simulink model "case_1_lead_veh_sudden_stop_25a"  (R2025b)
settings: Solver=VariableStepAuto  StartTime=0.0  StopTime=10.0  RelTol=1e-3
settings Model: Creator=admin  LastModifiedBy=admin

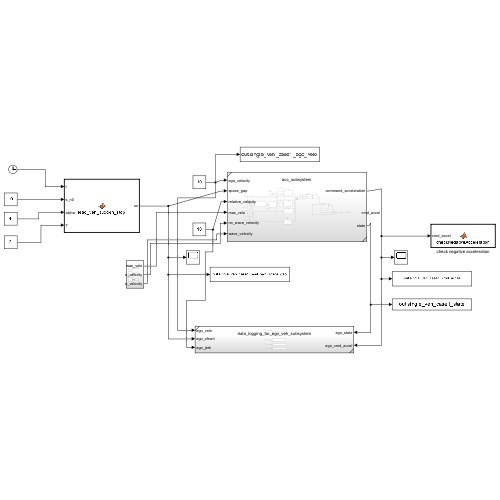
[thumbnail: Simulink's stored preview of the top-level diagram]
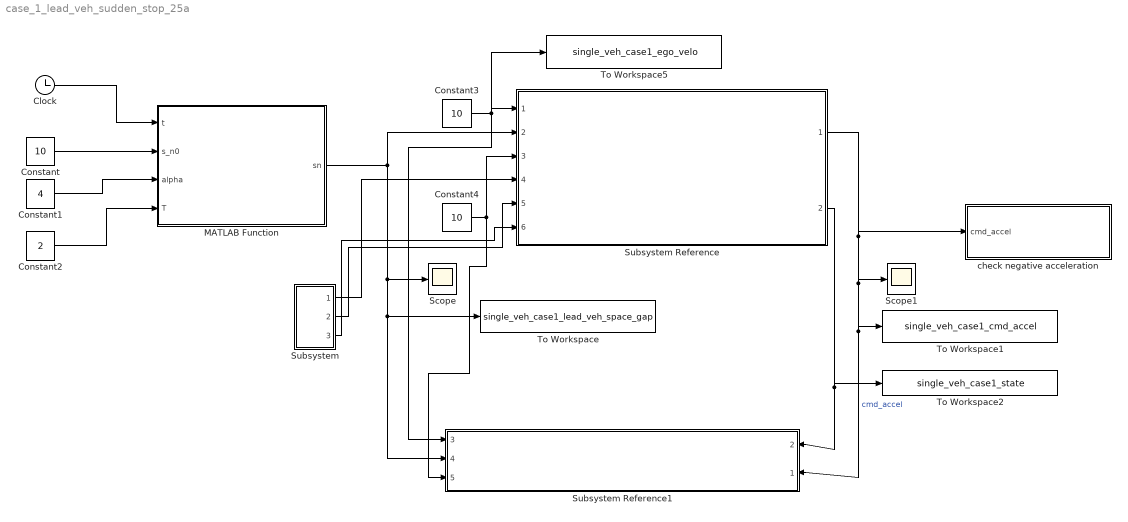
== system case_1_lead_veh_sudden_stop_25a ==
  Clock : Clock
  Constant : Constant  Value=10
  Constant1 : Constant  Value=4
  Constant2 : Constant  Value=2
  Constant3 : Constant  Value=10
  Constant4 : Constant  Value=10
  MATLAB Function : MATLAB Function  TreatAsAtomicUnit=on
  Scope : Scope
      settings: ActiveDisplayYMinimum=-2.4454295544676485  ActiveDisplayYMaximum=12.748398570532352
  Scope1 : Scope
      settings: ActiveDisplayYMinimum=-4  ActiveDisplayYMaximum=-2
  Subsystem : Subsystem
  Subsystem Reference : Subsystem  ReferencedSubsystem=acc_subsystem
  Subsystem Reference1 : Subsystem  ReferencedSubsystem=data_logging_for_ego_veh_subsystem
      settings: PortSchema="{\"entries\":[{\"content\":{\"sides\":[{\"content\":{\"connectorIds\":[\"In3\",\"In4\",\"In5\"]},\"type\":\"ConnectorPlacement.EquallySpacedRectSide\",\"uuid\":\"0b96bcaa-a470-46c9-9268-f4bd6b1035a8\"},{\"content\":{\"connectorIds\":[\"In2\",\"In1\"],\"side\":\"RIGHT\"},\"type\":\"ConnectorPlacement.EquallySpacedRectSide\",\"uuid\":\"8e49005a-1e53-4e76-b163-50df0eb9f2cc\"},{\"content\":{\"side\":\"TOP\"},\"type\":\"ConnectorPlacement.EquallySpacedRectSide\",\"uuid\":\"3ff4af65-efca-4a64-9b7f-f479498e89e2\"}]},\"type\":\"ConnectorPlacement.EquallySpacedConnector\",\"uuid\":\"f10caef7-9599-4d5c-a8fd-3eb49f6fcaa8\"}],\"packageUris\":[\"http://schema.mathworks.com/mf0/Connector/R2020b\"],\"version\":\"1.0\"}"
  To Workspace : ToWorkspace  VariableName=single_veh_case1_lead_veh_space_gap  SaveFormat=Structure With Time  SampleTime=-1
  To Workspace1 : ToWorkspace  VariableName=single_veh_case1_cmd_accel  SaveFormat=Structure With Time  SampleTime=-1
  To Workspace2 : ToWorkspace  VariableName=single_veh_case1_state  SaveFormat=Structure With Time  SampleTime=-1
  To Workspace5 : ToWorkspace  VariableName=single_veh_case1_ego_velo  SaveFormat=Structure With Time  SampleTime=-1
  check negative acceleration : MATLAB Function  TreatAsAtomicUnit=on
  wires:
  Clock/1 -> MATLAB Function/1(t)
  Constant/1 -> MATLAB Function/2(s_n0)
  Constant1/1 -> MATLAB Function/3(alpha)
  Constant2/1 -> MATLAB Function/4(T)
  Subsystem Reference/1 -> check negative acceleration/1(cmd_accel), Subsystem Reference1/1, To Workspace1/1, Scope1/1  "cmd_accel"
  Constant3/1 -> Subsystem Reference1/3, To Workspace5/1, Subsystem Reference/1
  MATLAB Function/1(sn) -> To Workspace/1, Subsystem Reference1/4, Scope/1, Subsystem Reference/2
  Subsystem Reference/2 -> Subsystem Reference1/2, To Workspace2/1
  Constant4/1 -> Subsystem Reference1/5, Subsystem Reference/3
  Subsystem/1(max_velo) -> Subsystem Reference/4
  Subsystem/2(no_wave_velocity) -> Subsystem Reference/5
  Subsystem/3(wave_velocity) -> Subsystem Reference/6

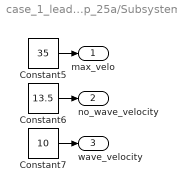
== system case_1_lead_veh_sudden_stop_25a/Subsystem ==
  Constant5 : Constant  Value=35
  Constant6 : Constant  Value=13.5
  Constant7 : Constant  Value=10
  max_velo : Outport
  no_wave_velocity : Outport  Port=2
  wave_velocity : Outport  Port=3
  wires:
  Constant7/1 -> wave_velocity/1
  Constant6/1 -> no_wave_velocity/1
  Constant5/1 -> max_velo/1

== matlab function case_1_lead_veh_sudden_stop_25a/MATLAB Function ==
  data: t input; sn output; s_n0 input; alpha input; T input
function sn = lead_veh_sudden_stop(t, s_n0, alpha, T)
    if t < T
        sn = s_n0;
    else
        sn = max(-alpha * s_n0, 0);
    end
end

== matlab function case_1_lead_veh_sudden_stop_25a/check negative acceleration ==
  data: cmd_accel input
function checkNegativeAcceleration(cmd_accel)
%#codegen
coder.extrinsic('disp', 'sprintf');

if cmd_accel >= 0
    msg = sprintf('Error: Positive command acceleration: %.3f, should be negative', ...
                  cmd_accel);
    disp(msg);
end
end
